simulink model "RefModel_GroundStation"  (R2020b)
settings: Solver=FixedStepAuto  StartTime=0.0  StopTime=150  FixedStep=Ts_GroundStation.Ts_base  RelTol=1e-3
values from neighbouring files (symbols this model uses):
  CMD_AirStandBy = STRUCT_mavlink_msg_id_command_long    [INIT_GROUNDSTATION.m]
  CMD_CamTriggDist = STRUCT_mavlink_msg_id_command_long    [INIT_GROUNDSTATION.m]
  CMD_Continue = STRUCT_mavlink_msg_id_command_long    [INIT_GROUNDSTATION.m]
  CMD_Fix2Rotor = STRUCT_mavlink_msg_id_command_long    [INIT_GROUNDSTATION.m]
  CMD_GoHome = STRUCT_mavlink_msg_id_command_long    [INIT_GROUNDSTATION.m]
  CMD_GoIntoPath = STRUCT_mavlink_msg_id_command_long    [INIT_GROUNDSTATION.m]
  CMD_GroundStandBy = STRUCT_mavlink_msg_id_command_long    [INIT_GROUNDSTATION.m]
  CMD_HoverAdjust = STRUCT_mavlink_msg_id_command_long    [INIT_GROUNDSTATION.m]
  CMD_LandStart = STRUCT_mavlink_msg_id_command_long    [INIT_GROUNDSTATION.m]
  CMD_ReGoIntoPath = STRUCT_mavlink_msg_id_command_long    [INIT_GROUNDSTATION.m]
  CMD_StartProfile = STRUCT_mavlink_msg_id_command_long    [INIT_GROUNDSTATION.m]
  CMD_SwitchAltitude = STRUCT_mavlink_msg_id_command_long    [INIT_GROUNDSTATION.m]
  CMD_TakeOff = STRUCT_mavlink_msg_id_command_long    [INIT_GROUNDSTATION.m]
  TASK_PARAM_V1000 = Simulink.Bus.createMATLABStruct('BUS_TASK_PATH_AlgoParam')    [INIT_Task.m]    (also in INIT_TaskManage.m)
undefined symbols (not defined in the file or in its folder): distBack, distFront, distLeft, distRight, ENUM_FlightTaskMode, flightTaskMode, groundspeedCmd, headingCmd, heightCmd, isRemoteConnected, isStationConnected, maxClimbSpeed, nBack, nFront, nLeft, nRight, stationLostTimeSec, STRUCT_mavlink_mission_item_def_ARRAY, TASK_SET, Ts_GroundStation, unlock
settings Model: PauseTimes=0  Creator=sl  LastModifiedBy=sl
settings DataIOCC: SaveOutput=off  SaveTime=off  ReturnWorkspaceOutputs=off
settings DebuggingCC: InheritedTsInSrcMsg=none  UnderSpecifiedDimensionMsg=warning  ArithmeticOperatorsInVariantConditions=warning
settings SFSimCC: CustomCodeUndefinedFunction=UseInterfaceOnly
settings GRTTargetCC: CombineOutputUpdateFcns=off  MatFileLogging=off

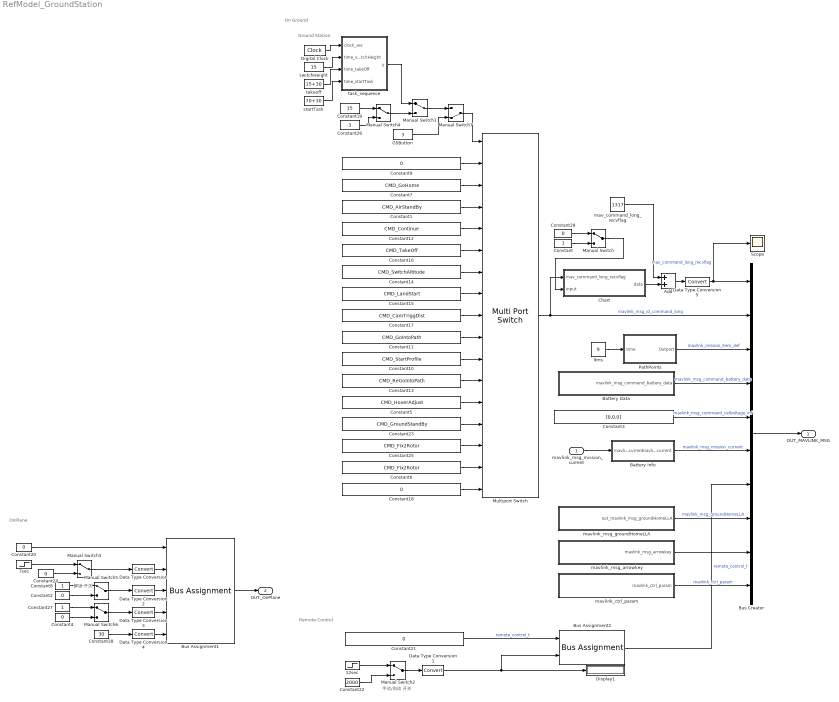
== system RefModel_GroundStation ==
  note: 手动/自动 开关
  note: Ground Station
  note: Remote Control
  note: OnPlane
  note: On Ground
  note: 解锁 开关
  mavlink_msg_mission_current : Inport  OutDataTypeStr=Bus: mavlink_msg_mission_current  BusOutputAsStruct=on
  12sec : Step  Time=12+30  Before=2000  After=1000  SampleTime=Ts_GroundStation.Ts_base  mask(DiscretizedSource){}
      mask init:
      | %zoh
  7sec : Step  Time=7+30  SampleTime=Ts_GroundStation.Ts_base  mask(DiscretizedSource){}
      mask init:
      | %zoh
  9ms : Constant  Value=9
  Add : Sum
  Battery Data : Subsystem
  Battery Info : Subsystem
  Bus Assignment1 : BusAssignment  AssignedSignals=unlock,isRemoteConnected,isStationConnected,stationLostTimeSec
  Bus Assignment2 : BusAssignment  AssignedSignals=chG_Mag
  Bus Creator : BusCreator  Inputs=10  OutDataTypeStr=Bus: BUS_MAVLINK_TO_FIRM  NonVirtualBus=on
  Chart : Stateflow chart  TreatAsAtomicUnit=on
  Constant : Constant
  Constant1 : Constant  Value=CMD_AirStandBy  OutDataTypeStr=Bus: mavlink_msg_id_command_long
  Constant10 : Constant  Value=CMD_StartProfile  OutDataTypeStr=Bus: mavlink_msg_id_command_long
  Constant11 : Constant  Value=CMD_GoIntoPath  OutDataTypeStr=Bus: mavlink_msg_id_command_long
  Constant12 : Constant  Value=CMD_Continue  OutDataTypeStr=Bus: mavlink_msg_id_command_long
  Constant13 : Constant  Value=CMD_ReGoIntoPath  OutDataTypeStr=Bus: mavlink_msg_id_command_long
  Constant14 : Constant  Value=CMD_SwitchAltitude  OutDataTypeStr=Bus: mavlink_msg_id_command_long
  Constant15 : Constant  Value=CMD_LandStart  OutDataTypeStr=Bus: mavlink_msg_id_command_long
  Constant16 : Constant  Value=CMD_TakeOff  OutDataTypeStr=Bus: mavlink_msg_id_command_long
  Constant17 : Constant  Value=CMD_CamTriggDist  OutDataTypeStr=Bus: mavlink_msg_id_command_long
  Constant18 : Constant  Value=0  OutDataTypeStr=Bus: mavlink_msg_id_command_long
  Constant19 : Constant  Value=15
  Constant{2,4,24,29} (4 alike) : Constant  Value=0
  Constant20 : Constant  Value=0  OutDataTypeStr=Bus: BUS_ONPLANE_FEEDBACK
  Constant21 : Constant  Value=0  OutDataTypeStr=Bus: remote_control_t
  Constant22 : Constant  Value=2000
  Constant23 : Constant  Value=CMD_GroundStandBy  OutDataTypeStr=Bus: mavlink_msg_id_command_long
  Constant25 : Constant  Value=CMD_Fix2Rotor  OutDataTypeStr=Bus: mavlink_msg_id_command_long
  Constant26 : Constant  Value=3
  Constant27 : Constant
  Constant28 : Constant  Value=30
  Constant3 : Constant  Value=[0,0,0]  OutDataTypeStr=Bus: mavlink_msg_command_cellvoltage_inf
  Constant5 : Constant  Value=CMD_HoverAdjust  OutDataTypeStr=Bus: mavlink_msg_id_command_long
  Constant6 : Constant  Value=CMD_Fix2Rotor  OutDataTypeStr=Bus: mavlink_msg_id_command_long
  Constant7 : Constant  Value=CMD_GoHome  OutDataTypeStr=Bus: mavlink_msg_id_command_long
  Constant8 : Constant
  Constant9 : Constant  Value=0  OutDataTypeStr=Bus: mavlink_msg_id_command_long
  Data Type Conversion{,1..5} (6 alike) : DataTypeConversion
  Digital Clock : DigitalClock  SampleTime=-1
  Display1 : Display
  GSButton : Constant  Value=3
  Manual Switch{,1..6} (7 alike) : ManualSwitch
  Manual Switch7 : ManualSwitch  CurrentSetting=0
  Multiport Switch : MultiPortSwitch  Inputs=15  DataPortForDefault=Additional data port  DiagnosticForDefault=Warning
  PathPoints : Subsystem
  Scope : Scope
  mav_command_long_recvflag : Constant  Value=1317
  mavlink_ctrl_param : Subsystem
  mavlink_msg_arrowkey : Subsystem
  mavlink_msg_groundHomeLLA : Subsystem
  startTask : Constant  Value=70+30
  switchHeight : Constant  Value=15
  takeoff : Constant  Value=15+30
  task_sequence : MATLAB Function  TreatAsAtomicUnit=on
  OUT_MAVLINK_MSG : Outport  OutDataTypeStr=Bus: BUS_MAVLINK_TO_FIRM  BusOutputAsStruct=on
  OUT_OnPlane : Outport  Port=2  OutDataTypeStr=Bus: BUS_ONPLANE_FEEDBACK
  wires:
  Bus Creator/1 -> OUT_MAVLINK_MSG/1
  Bus Assignment1/1 -> OUT_OnPlane/1
  Battery Info/1(mavlink_msg_mission_current) -> Bus Creator/6  "mavlink_msg_mission_current"
  Constant3/1 -> Bus Creator/5  "mavlink_msg_command_cellvoltage_inf"
  PathPoints/1(Outport) -> Bus Creator/3  "mavlink_mission_item_def"
  Multiport Switch/1 -> Chart/1(mav_command_long_recvflag), Bus Creator/2  "mavlink_msg_id_command_long"
  Constant20/1 -> Bus Assignment1/1
  Constant21/1 -> Bus Assignment2/1  "remote_control_t"
  Bus Assignment2/1 -> Bus Creator/7  "remote_control_t"
  Data Type Conversion1/1 -> Bus Assignment2/2, Display1/1
  Manual Switch2/1 -> Data Type Conversion1/1
  12sec/1 -> Manual Switch2/1
  Constant22/1 -> Manual Switch2/2
  Constant24/1 -> Manual Switch3/2
  Data Type Conversion/1 -> Bus Assignment1/2
  7sec/1 -> Manual Switch3/1
  Manual Switch3/1 -> Data Type Conversion/1
  Battery Data/1(mavlink_msg_command_battery_data) -> Bus Creator/4  "mavlink_msg_command_battery_data"
  Data Type Conversion2/1 -> Bus Assignment1/3
  Data Type Conversion3/1 -> Bus Assignment1/4
  Data Type Conversion4/1 -> Bus Assignment1/5
  Constant28/1 -> Data Type Conversion4/1
  Manual Switch5/1 -> Data Type Conversion2/1
  Constant8/1 -> Manual Switch5/1
  Constant2/1 -> Manual Switch5/2
  Constant4/1 -> Manual Switch6/2
  Constant27/1 -> Manual Switch6/1
  Manual Switch6/1 -> Data Type Conversion3/1
  9ms/1 -> PathPoints/1(time)
  Constant29/1 -> Manual Switch/1
  Constant/1 -> Manual Switch/2
  Manual Switch/1 -> Chart/2(input)
  Data Type Conversion5/1 -> Scope/1, Bus Creator/1  "mav_command_long_recvflag"
  mavlink_msg_groundHomeLLA/1(out_mavlink_msg_groundHomeLLA) -> Bus Creator/8  "mavlink_msg_groundHomeLLA"
  Chart/1(data) -> Add/2
  Add/1 -> Data Type Conversion5/1
  mav_command_long_recvflag/1 -> Add/1
  mavlink_msg_arrowkey/1(mavlink_msg_arrowkey) -> Bus Creator/9
  mavlink_msg_mission_current/1 -> Battery Info/1("mavlink_msg_mission_current ")
  mavlink_ctrl_param/1(mavlink_ctrl_param) -> Bus Creator/10  "mavlink_ctrl_param"
  Constant15/1 -> Multiport Switch/8
  Constant16/1 -> Multiport Switch/6
  Constant19/1 -> Manual Switch4/1
  Constant1/1 -> Multiport Switch/4
  Manual Switch1/1 -> Manual Switch7/1
  Constant17/1 -> Multiport Switch/9
  GSButton/1 -> Manual Switch7/2
  Digital Clock/1 -> task_sequence/1(clock_sec)
  Constant26/1 -> Manual Switch4/2
  Constant10/1 -> Multiport Switch/11
  startTask/1 -> task_sequence/4(time_startTask)
  Constant9/1 -> Multiport Switch/2
  takeoff/1 -> task_sequence/3(time_takeOff)
  Constant13/1 -> Multiport Switch/12
  Constant7/1 -> Multiport Switch/3
  Constant18/1 -> Multiport Switch/17
  Constant12/1 -> Multiport Switch/5
  Constant5/1 -> Multiport Switch/13
  Constant25/1 -> Multiport Switch/15
  Constant14/1 -> Multiport Switch/7
  Manual Switch7/1 -> Multiport Switch/1
  Constant6/1 -> Multiport Switch/16
  task_sequence/1(y) -> Manual Switch1/1
  Constant23/1 -> Multiport Switch/14
  Manual Switch4/1 -> Manual Switch1/2
  Constant11/1 -> Multiport Switch/10
  switchHeight/1 -> task_sequence/2(time_switchHeight)

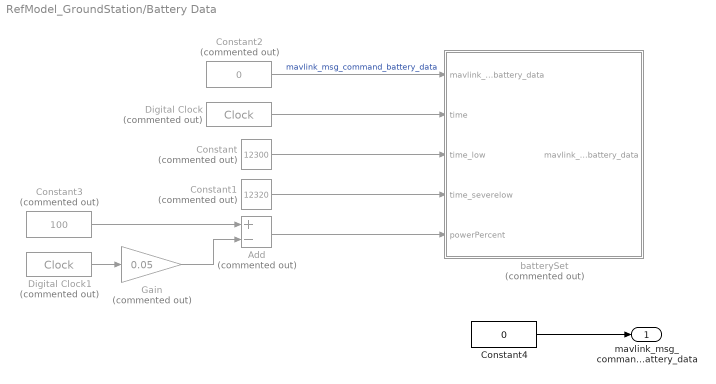
== system RefModel_GroundStation/Battery Data ==
  Add : Sum  Commented=on  Inputs=+-
  Constant : Constant  Commented=on  Value=12300
  Constant1 : Constant  Commented=on  Value=12320
  Constant2 : Constant  Commented=on  Value=0  OutDataTypeStr=Bus: mavlink_msg_command_battery_data
  Constant3 : Constant  Commented=on  Value=100
  Constant4 : Constant  Value=0  OutDataTypeStr=Bus: mavlink_msg_command_battery_data
  Digital Clock : DigitalClock  Commented=on  SampleTime=-1
  Digital Clock1 : DigitalClock  Commented=on  SampleTime=-1
  Gain : Gain  Commented=on  Gain=0.05
  batterySet : MATLAB Function  Commented=on  TreatAsAtomicUnit=on
  mavlink_msg_command_battery_data : Outport
  wires:
  Constant2/1 -> batterySet/1("mavlink_msg_command_battery_data ")  "mavlink_msg_command_battery_data"
  Constant4/1 -> mavlink_msg_command_battery_data/1
  Digital Clock/1 -> batterySet/2(time)
  Constant/1 -> batterySet/3(time_low)
  Constant1/1 -> batterySet/4(time_severelow)
  Add/1 -> batterySet/5(powerPercent)
  Constant3/1 -> Add/1
  Digital Clock1/1 -> Gain/1
  Gain/1 -> Add/2

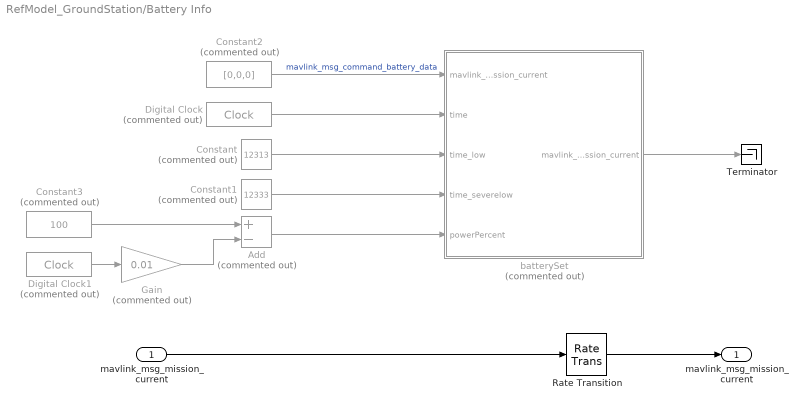
== system RefModel_GroundStation/Battery Info ==
  "mavlink_msg_mission_current " : Inport
  Add : Sum  Commented=on  Inputs=+-
  Constant : Constant  Commented=on  Value=12313
  Constant1 : Constant  Commented=on  Value=12333
  Constant2 : Constant  Commented=on  Value=[0,0,0]  OutDataTypeStr=Bus: mavlink_msg_mission_current
  Constant3 : Constant  Commented=on  Value=100
  Digital Clock : DigitalClock  Commented=on  SampleTime=-1
  Digital Clock1 : DigitalClock  Commented=on  SampleTime=-1
  Gain : Gain  Commented=on  Gain=0.01
  Rate Transition : RateTransition
  Terminator : Terminator
  batterySet : MATLAB Function  Commented=on  TreatAsAtomicUnit=on
  mavlink_msg_mission_current : Outport
  wires:
  Gain/1 -> Add/2
  Digital Clock1/1 -> Gain/1
  Constant3/1 -> Add/1
  Add/1 -> batterySet/5(powerPercent)
  Constant1/1 -> batterySet/4(time_severelow)
  Constant/1 -> batterySet/3(time_low)
  Digital Clock/1 -> batterySet/2(time)
  batterySet/1(mavlink_msg_mission_current) -> Terminator/1
  Constant2/1 -> batterySet/1("mavlink_msg_mission_current ")  "mavlink_msg_command_battery_data"
  Rate Transition/1 -> mavlink_msg_mission_current/1
  "mavlink_msg_mission_current "/1 -> Rate Transition/1

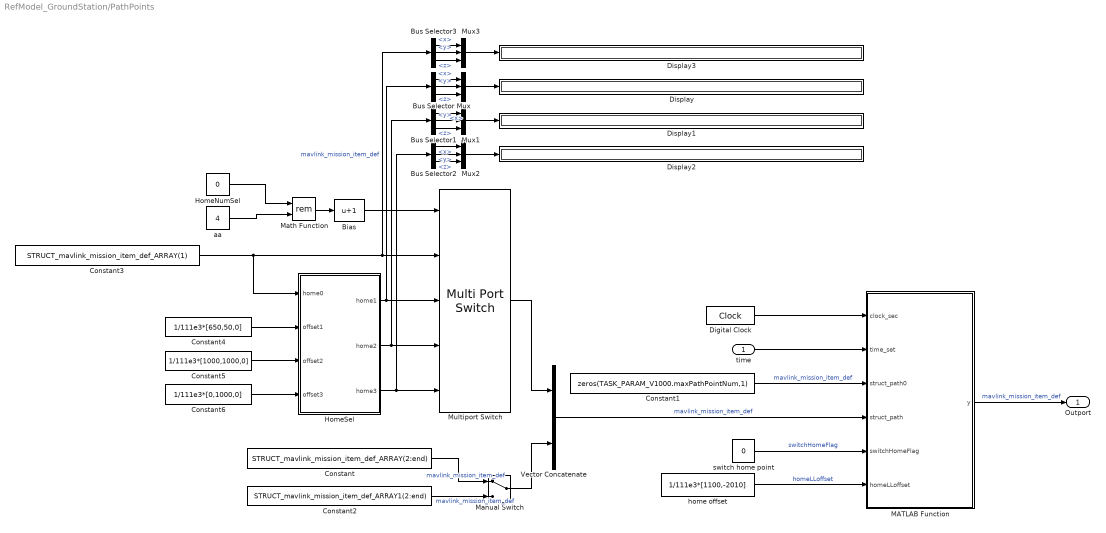
== system RefModel_GroundStation/PathPoints ==
  time : Inport
  Bias : Bias  Bias=1
  Bus Selector{,1..3} (4 alike) : BusSelector  OutputSignals=x,y,z
  Constant : Constant  Value=STRUCT_mavlink_mission_item_def_ARRAY(2:end)  OutDataTypeStr=Bus: mavlink_mission_item_def
  Constant1 : Constant  Value=zeros(TASK_PARAM_V1000.maxPathPointNum,1)  OutDataTypeStr=Bus: mavlink_mission_item_def
  Constant2 : Constant  Value=STRUCT_mavlink_mission_item_def_ARRAY1(2:end)  OutDataTypeStr=Bus: mavlink_mission_item_def
  Constant3 : Constant  Value=STRUCT_mavlink_mission_item_def_ARRAY(1)  OutDataTypeStr=Bus: mavlink_mission_item_def
  Constant4 : Constant  Value=1/111e3*[650,50,0]
  Constant5 : Constant  Value=1/111e3*[1000,1000,0]
  Constant6 : Constant  Value=1/111e3*[0,1000,0]
  Digital Clock : DigitalClock  SampleTime=-1
  Display{,1..3} (4 alike) : Display
  HomeNumSel : Constant  Value=0
  HomeSel : MATLAB Function  TreatAsAtomicUnit=on
  MATLAB Function : MATLAB Function  TreatAsAtomicUnit=on
  Manual Switch : ManualSwitch
  Math Function : Math  Operator=rem  SaturateOnIntegerOverflow=on
  Multiport Switch : MultiPortSwitch  Inputs=4
  Mux{,1..3} (4 alike) : Mux  Inputs=3
  Vector Concatenate : Concatenate
  aa : Constant  Value=4
  home offset : Constant  Value=1/111e3*[1100,-2010]
  switch home point : Constant  Value=0
  Outport : Outport
  wires:
  MATLAB Function/1(y) -> Outport/1  "mavlink_mission_item_def"
  Digital Clock/1 -> MATLAB Function/1(clock_sec)
  time/1 -> MATLAB Function/2(time_set)
  Constant1/1 -> MATLAB Function/3(struct_path0)  "mavlink_mission_item_def"
  Vector Concatenate/1 -> MATLAB Function/4(struct_path)  "mavlink_mission_item_def"
  switch home point/1 -> MATLAB Function/5(switchHomeFlag)  "switchHomeFlag"
  home offset/1 -> MATLAB Function/6(homeLLoffset)  "homeLLoffset"
  Constant/1 -> Manual Switch/1  "mavlink_mission_item_def"
  HomeNumSel/1 -> Math Function/1
  Multiport Switch/1 -> Vector Concatenate/1
  Constant3/1 -> HomeSel/1(home0), Bus Selector3/1, Multiport Switch/2  "mavlink_mission_item_def"
  Constant4/1 -> HomeSel/2(offset1)
  Constant5/1 -> HomeSel/3(offset2)
  Constant6/1 -> HomeSel/4(offset3)
  HomeSel/3(home3) -> Bus Selector2/1, Multiport Switch/5
  HomeSel/2(home2) -> Bus Selector1/1, Multiport Switch/4
  HomeSel/1(home1) -> Bus Selector/1, Multiport Switch/3
  Bus Selector/1 -> Mux/1  "<x>"
  Bus Selector/2 -> Mux/2  "<y>"
  Bus Selector/3 -> Mux/3  "<z>"
  Mux/1 -> Display/1
  Mux1/1 -> Display1/1
  Bus Selector1/3 -> Mux1/3  "<z>"
  Bus Selector1/2 -> Mux1/2  "<y>"
  Bus Selector1/1 -> Mux1/1  "<x>"
  Bus Selector2/1 -> Mux2/1  "<x>"
  Bus Selector2/2 -> Mux2/2  "<y>"
  Bus Selector2/3 -> Mux2/3  "<z>"
  Mux2/1 -> Display2/1
  Mux3/1 -> Display3/1
  Bus Selector3/3 -> Mux3/3  "<z>"
  Bus Selector3/2 -> Mux3/2  "<y>"
  Bus Selector3/1 -> Mux3/1  "<x>"
  Constant2/1 -> Manual Switch/2  "mavlink_mission_item_def"
  Manual Switch/1 -> Vector Concatenate/2
  Math Function/1 -> Bias/1
  aa/1 -> Math Function/2
  Bias/1 -> Multiport Switch/1

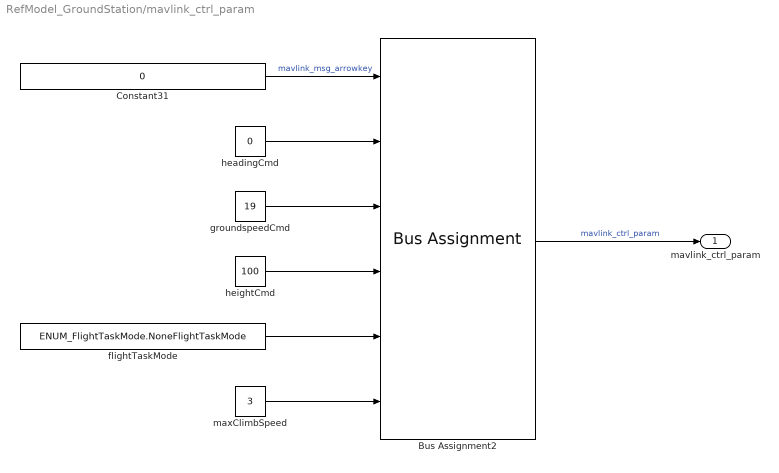
== system RefModel_GroundStation/mavlink_ctrl_param ==
  Bus Assignment2 : BusAssignment  AssignedSignals=headingCmd,groundspeedCmd,heightCmd,flightTaskMode,maxClimbSpeed
  Constant31 : Constant  Value=0  OutDataTypeStr=Bus: mavlink_ctrl_param
  flightTaskMode : Constant  Value=ENUM_FlightTaskMode.NoneFlightTaskMode
  groundspeedCmd : Constant  Value=19
  headingCmd : Constant  Value=0
  heightCmd : Constant  Value=100
  maxClimbSpeed : Constant  Value=3
  mavlink_ctrl_param : Outport
  wires:
  Constant31/1 -> Bus Assignment2/1  "mavlink_msg_arrowkey"
  Bus Assignment2/1 -> mavlink_ctrl_param/1  "mavlink_ctrl_param"
  headingCmd/1 -> Bus Assignment2/2
  groundspeedCmd/1 -> Bus Assignment2/3
  heightCmd/1 -> Bus Assignment2/4
  maxClimbSpeed/1 -> Bus Assignment2/6
  flightTaskMode/1 -> Bus Assignment2/5

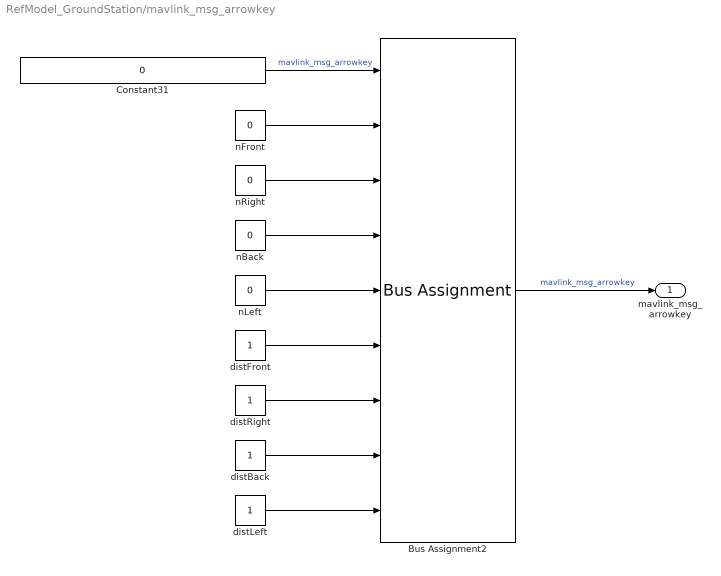
== system RefModel_GroundStation/mavlink_msg_arrowkey ==
  Bus Assignment2 : BusAssignment  AssignedSignals=nFront,nRight,nBack,nLeft,distFront,distRight,distBack,distLeft
  Constant31 : Constant  Value=0  OutDataTypeStr=Bus: BUS_TASK_ARROWKEY
  distBack : Constant
  distFront : Constant
  distLeft : Constant
  distRight : Constant
  nBack : Constant  Value=0
  nFront : Constant  Value=0
  nLeft : Constant  Value=0
  nRight : Constant  Value=0
  mavlink_msg_arrowkey : Outport
  wires:
  Bus Assignment2/1 -> mavlink_msg_arrowkey/1  "mavlink_msg_arrowkey"
  Constant31/1 -> Bus Assignment2/1  "mavlink_msg_arrowkey"
  nFront/1 -> Bus Assignment2/2
  nRight/1 -> Bus Assignment2/3
  nBack/1 -> Bus Assignment2/4
  nLeft/1 -> Bus Assignment2/5
  distFront/1 -> Bus Assignment2/6
  distRight/1 -> Bus Assignment2/7
  distBack/1 -> Bus Assignment2/8
  distLeft/1 -> Bus Assignment2/9

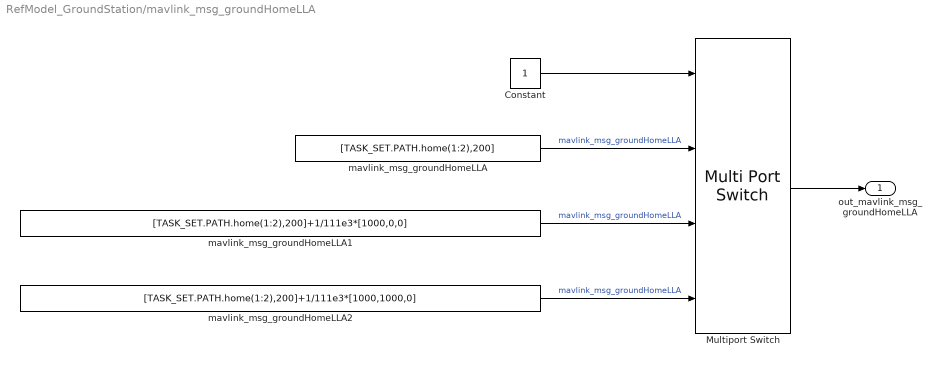
== system RefModel_GroundStation/mavlink_msg_groundHomeLLA ==
  Constant : Constant
  Multiport Switch : MultiPortSwitch
  mavlink_msg_groundHomeLLA : Constant  Value=[TASK_SET.PATH.home(1:2),200]  OutDataTypeStr=Inherit: Inherit via back propagation
  mavlink_msg_groundHomeLLA1 : Constant  Value=[TASK_SET.PATH.home(1:2),200]+1/111e3*[1000,0,0]  OutDataTypeStr=Inherit: Inherit via back propagation
  mavlink_msg_groundHomeLLA2 : Constant  Value=[TASK_SET.PATH.home(1:2),200]+1/111e3*[1000,1000,0]  OutDataTypeStr=Inherit: Inherit via back propagation
  out_mavlink_msg_groundHomeLLA : Outport
  wires:
  mavlink_msg_groundHomeLLA/1 -> Multiport Switch/2  "mavlink_msg_groundHomeLLA"
  Multiport Switch/1 -> out_mavlink_msg_groundHomeLLA/1
  Constant/1 -> Multiport Switch/1
  mavlink_msg_groundHomeLLA1/1 -> Multiport Switch/3  "mavlink_msg_groundHomeLLA"
  mavlink_msg_groundHomeLLA2/1 -> Multiport Switch/4  "mavlink_msg_groundHomeLLA"

== matlab function RefModel_GroundStation/task_sequence ==
  data: clock_sec input; time_switchHeight input; y output; time_takeOff input; time_startTask input
function y = fcn(clock_sec, time_switchHeight, time_takeOff, time_startTask)
if clock_sec >= time_switchHeight && clock_sec < time_takeOff
    y = 6;
elseif clock_sec >= time_takeOff && clock_sec < time_startTask
    y = 5;
elseif clock_sec >= time_startTask
    y = 4;
else
    y = 1;
end

== matlab function RefModel_GroundStation/Battery Data/batterySet ==
  data: mavlink_msg_command_battery_data input Bus: mavlink_msg_command_battery_data; mavlink_msg_command_battery_data output size=3; time input; time_low input; time_severelow input; powerPercent input
function mavlink_msg_command_battery_data  = fcn(mavlink_msg_command_battery_data, time, time_low, time_severelow,powerPercent)
if time > time_low && time <= time_severelow
    mavlink_msg_command_battery_data.battery(1).lifePercent = uint8(19);
    mavlink_msg_command_battery_data.battery(2).lifePercent = uint8(20);
    mavlink_msg_command_battery_data.battery(3).lifePercent = uint8(22);
elseif time > time_severelow
    mavlink_msg_command_battery_data.battery(1).lifePercent = uint8(6);
    mavlink_msg_command_battery_data.battery(2).lifePercent = uint8(4);
    mavlink_msg_command_battery_data.battery(3).lifePercent = uint8(6);
elseif time < 10
    mavlink_msg_command_battery_data.battery(1).lifePercent = uint8(0);
    mavlink_msg_command_battery_data.battery(2).lifePercent = uint8(0);
    mavlink_msg_command_battery_data.battery(3).lifePercent = uint8(0);
else
    mavlink_msg_command_battery_data.battery(1).lifePercent = uint8(powerPercent);
    mavlink_msg_command_battery_data.battery(2).lifePercent = uint8(powerPercent);
    mavlink_msg_command_battery_data.battery(3).lifePercent = uint8(powerPercent);
end

== matlab function RefModel_GroundStation/PathPoints/MATLAB Function ==
  data: clock_sec input; y output Bus: mavlink_mission_item_def; time_set input; struct_path0 input Bus: mavlink_mission_item_def; struct_path input Bus: mavlink_mission_item_def; switchHomeFlag input; homeLLoffset input
function y = fcn(clock_sec,time_set,struct_path0,struct_path, switchHomeFlag, homeLLoffset)
if clock_sec > time_set 
    y = struct_path;
    if switchHomeFlag
        y(1).x = y(1).x + homeLLoffset(1);
        y(1).y = y(1).y + homeLLoffset(2);
    end
else
    y = struct_path0;
end

== stateflow chart RefModel_GroundStation/Chart ==
  state State
    en:
    data = 0;
    du:
    data = data + input;
    if hasChanged(mav_command_long_recvflag.command)
    data = data + 1;
    end
  (default) -> State
  data: mav_command_long_recvflag input; data output; input input

== matlab function RefModel_GroundStation/Battery Info/batterySet ==
  data: mavlink_msg_mission_current input Bus: mavlink_msg_mission_current; mavlink_msg_mission_current output size=3; time input; time_low input; time_severelow input; powerPercent input
function mavlink_msg_mission_current  = fcn(mavlink_msg_mission_current, time, time_low, time_severelow,powerPercent)
if time > time_low && time <= time_severelow
    mavlink_msg_mission_current(1).remaining = int8(19);
    mavlink_msg_mission_current(2).remaining = int8(20);
    mavlink_msg_mission_current(3).remaining = int8(22);
elseif time > time_severelow
    mavlink_msg_mission_current(1).remaining = int8(6);
    mavlink_msg_mission_current(2).remaining = int8(4);
    mavlink_msg_mission_current(3).remaining = int8(6);
elseif time < 10
    mavlink_msg_mission_current(1).remaining = int8(0);
    mavlink_msg_mission_current(2).remaining = int8(0);
    mavlink_msg_mission_current(3).remaining = int8(0);
else
    mavlink_msg_mission_current(1).remaining = int8(powerPercent);
    mavlink_msg_mission_current(2).remaining = int8(powerPercent);
    mavlink_msg_mission_current(3).remaining = int8(powerPercent);
end

== matlab function RefModel_GroundStation/PathPoints/HomeSel ==
  data: home0 input Bus: mavlink_mission_item_def; home1 output Bus: mavlink_mission_item_def; offset1 input; offset2 input; home2 output Bus: mavlink_mission_item_def; offset3 input; home3 output Bus: mavlink_mission_item_def
function [home1,home2,home3] = fcn(home0, offset1, offset2, offset3)
home1 = home0;
home1.x = home0.x + offset1(1);
home1.y = home0.y + offset1(2);
home2 = home0;
home2.x = home0.x + offset2(1);
home2.y = home0.y + offset2(2);
home3 = home0;
home3.x = home0.x + offset3(1);
home3.y = home0.y + offset3(2);
